simulink model "gm_uz_ninephase_VSD_transformation"  (R2021b)
settings: Solver=FixedStepAuto  StartTime=0.0  StopTime=inf  RelTol=1e-3
undefined symbols (not defined in the file or in its folder): a, b, c
libraries: hdlsllib x90, simulink x32, hdlmdlgenlib x20, dspsigops x7
(part 3 of 6)

== system gm_uz_ninephase_VSD_transformation/abc_to_dq/Divide ==
  in0 : Inport  OutDataTypeStr=fixdt(1, 18, 16)  SampleTime=1e-10
  in1 : Inport  Port=2  OutDataTypeStr=fixdt(1, 27, 16)  SampleTime=1e-10
  globalSchedule : EnablePort  OutDataTypeStr=boolean
  Divide : Product  Inputs=**  OutDataTypeStr=fixdt(1, 27, 16)  SampleTime=1e-10
  HwModeRegister : Delay  DelayLength=double(1)  InitialCondition=0
  HwModeRegister1 : Delay  DelayLength=double(1)  InitialCondition=0
  PipelineRegister : Delay  DelayLength=double(1)  InitialCondition=0
  out0 : Outport  OutDataTypeStr=fixdt(1, 27, 16)  SampleTime=1e-10  InitialOutput=0
  wires:
  PipelineRegister/1 -> out0/1
  in0/1 -> HwModeRegister/1
  in1/1 -> HwModeRegister1/1
  Divide/1 -> PipelineRegister/1
  HwModeRegister/1 -> Divide/1
  HwModeRegister1/1 -> Divide/2

== system gm_uz_ninephase_VSD_transformation/abc_to_dq/Divide1 ==
  in0 : Inport  OutDataTypeStr=fixdt(1, 18, 16)  SampleTime=1e-10
  in1 : Inport  Port=2  OutDataTypeStr=fixdt(1, 27, 16)  SampleTime=1e-10
  globalSchedule : EnablePort  OutDataTypeStr=boolean
  Divide1 : Product  Inputs=**  OutDataTypeStr=fixdt(1, 27, 16)  SampleTime=1e-10
  HwModeRegister : Delay  DelayLength=double(1)  InitialCondition=0
  HwModeRegister1 : Delay  DelayLength=double(1)  InitialCondition=0
  PipelineRegister : Delay  DelayLength=double(1)  InitialCondition=0
  out0 : Outport  OutDataTypeStr=fixdt(1, 27, 16)  SampleTime=1e-10  InitialOutput=0
  wires:
  PipelineRegister/1 -> out0/1
  in0/1 -> HwModeRegister/1
  in1/1 -> HwModeRegister1/1
  Divide1/1 -> PipelineRegister/1
  HwModeRegister/1 -> Divide1/1
  HwModeRegister1/1 -> Divide1/2

== system gm_uz_ninephase_VSD_transformation/abc_to_dq/Divide11 ==
  in0 : Inport  OutDataTypeStr=fixdt(1, 18, 16)  SampleTime=1e-10
  in1 : Inport  Port=2  OutDataTypeStr=fixdt(1, 27, 18)  SampleTime=1e-10
  globalSchedule : EnablePort  OutDataTypeStr=boolean
  Divide1 : Product  Inputs=**  OutDataTypeStr=fixdt(1, 27, 18)  SampleTime=1e-10
  HwModeRegister : Delay  DelayLength=double(1)  InitialCondition=0
  HwModeRegister1 : Delay  DelayLength=double(1)  InitialCondition=0
  PipelineRegister : Delay  DelayLength=double(1)  InitialCondition=0
  out0 : Outport  OutDataTypeStr=fixdt(1, 27, 18)  SampleTime=1e-10  InitialOutput=0
  wires:
  PipelineRegister/1 -> out0/1
  in0/1 -> HwModeRegister/1
  in1/1 -> HwModeRegister1/1
  Divide1/1 -> PipelineRegister/1
  HwModeRegister/1 -> Divide1/1
  HwModeRegister1/1 -> Divide1/2

== system gm_uz_ninephase_VSD_transformation/abc_to_dq/Divide2 ==
  in0 : Inport  OutDataTypeStr=fixdt(1, 18, 16)  SampleTime=1e-10
  in1 : Inport  Port=2  OutDataTypeStr=fixdt(1, 27, 18)  SampleTime=1e-10
  globalSchedule : EnablePort  OutDataTypeStr=boolean
  Divide2 : Product  Inputs=**  OutDataTypeStr=fixdt(1, 27, 18)  SampleTime=1e-10
  HwModeRegister : Delay  DelayLength=double(1)  InitialCondition=0
  HwModeRegister1 : Delay  DelayLength=double(1)  InitialCondition=0
  PipelineRegister : Delay  DelayLength=double(1)  InitialCondition=0
  out0 : Outport  OutDataTypeStr=fixdt(1, 27, 18)  SampleTime=1e-10  InitialOutput=0
  wires:
  PipelineRegister/1 -> out0/1
  in0/1 -> HwModeRegister/1
  in1/1 -> HwModeRegister1/1
  Divide2/1 -> PipelineRegister/1
  HwModeRegister/1 -> Divide2/1
  HwModeRegister1/1 -> Divide2/2

== system gm_uz_ninephase_VSD_transformation/abc_to_dq/Divide21 ==
  in0 : Inport  OutDataTypeStr=fixdt(1, 18, 16)  SampleTime=1e-10
  in1 : Inport  Port=2  OutDataTypeStr=fixdt(1, 27, 16)  SampleTime=1e-10
  globalSchedule : EnablePort  OutDataTypeStr=boolean
  Divide2 : Product  Inputs=**  OutDataTypeStr=fixdt(1, 27, 16)  SampleTime=1e-10
  HwModeRegister : Delay  DelayLength=double(1)  InitialCondition=0
  HwModeRegister1 : Delay  DelayLength=double(1)  InitialCondition=0
  PipelineRegister : Delay  DelayLength=double(1)  InitialCondition=0
  out0 : Outport  OutDataTypeStr=fixdt(1, 27, 16)  SampleTime=1e-10  InitialOutput=0
  wires:
  PipelineRegister/1 -> out0/1
  in0/1 -> HwModeRegister/1
  in1/1 -> HwModeRegister1/1
  Divide2/1 -> PipelineRegister/1
  HwModeRegister/1 -> Divide2/1
  HwModeRegister1/1 -> Divide2/2

== system gm_uz_ninephase_VSD_transformation/abc_to_dq/Divide3 ==
  in0 : Inport  OutDataTypeStr=fixdt(1, 18, 16)  SampleTime=1e-10
  in1 : Inport  Port=2  OutDataTypeStr=fixdt(1, 27, 18)  SampleTime=1e-10
  globalSchedule : EnablePort  OutDataTypeStr=boolean
  Divide3 : Product  Inputs=**  OutDataTypeStr=fixdt(1, 27, 18)  SampleTime=1e-10
  HwModeRegister : Delay  DelayLength=double(1)  InitialCondition=0
  HwModeRegister1 : Delay  DelayLength=double(1)  InitialCondition=0
  PipelineRegister : Delay  DelayLength=double(1)  InitialCondition=0
  out0 : Outport  OutDataTypeStr=fixdt(1, 27, 18)  SampleTime=1e-10  InitialOutput=0
  wires:
  PipelineRegister/1 -> out0/1
  in0/1 -> HwModeRegister/1
  in1/1 -> HwModeRegister1/1
  Divide3/1 -> PipelineRegister/1
  HwModeRegister/1 -> Divide3/1
  HwModeRegister1/1 -> Divide3/2

== system gm_uz_ninephase_VSD_transformation/abc_to_dq/Divide31 ==
  in0 : Inport  OutDataTypeStr=fixdt(1, 18, 16)  SampleTime=1e-10
  in1 : Inport  Port=2  OutDataTypeStr=fixdt(1, 27, 16)  SampleTime=1e-10
  globalSchedule : EnablePort  OutDataTypeStr=boolean
  Divide3 : Product  Inputs=**  OutDataTypeStr=fixdt(1, 27, 16)  SampleTime=1e-10
  HwModeRegister : Delay  DelayLength=double(1)  InitialCondition=0
  HwModeRegister1 : Delay  DelayLength=double(1)  InitialCondition=0
  PipelineRegister : Delay  DelayLength=double(1)  InitialCondition=0
  out0 : Outport  OutDataTypeStr=fixdt(1, 27, 16)  SampleTime=1e-10  InitialOutput=0
  wires:
  PipelineRegister/1 -> out0/1
  in0/1 -> HwModeRegister/1
  in1/1 -> HwModeRegister1/1
  Divide3/1 -> PipelineRegister/1
  HwModeRegister/1 -> Divide3/1
  HwModeRegister1/1 -> Divide3/2

== system gm_uz_ninephase_VSD_transformation/abc_to_dq/Divide4 ==
  in0 : Inport  OutDataTypeStr=fixdt(1, 18, 16)  SampleTime=1e-10
  in1 : Inport  Port=2  OutDataTypeStr=fixdt(1, 27, 18)  SampleTime=1e-10
  globalSchedule : EnablePort  OutDataTypeStr=boolean
  Divide : Product  Inputs=**  OutDataTypeStr=fixdt(1, 27, 18)  SampleTime=1e-10
  HwModeRegister : Delay  DelayLength=double(1)  InitialCondition=0
  HwModeRegister1 : Delay  DelayLength=double(1)  InitialCondition=0
  PipelineRegister : Delay  DelayLength=double(1)  InitialCondition=0
  out0 : Outport  OutDataTypeStr=fixdt(1, 27, 18)  SampleTime=1e-10  InitialOutput=0
  wires:
  PipelineRegister/1 -> out0/1
  in0/1 -> HwModeRegister/1
  in1/1 -> HwModeRegister1/1
  Divide/1 -> PipelineRegister/1
  HwModeRegister/1 -> Divide/1
  HwModeRegister1/1 -> Divide/2

== system gm_uz_ninephase_VSD_transformation/abc_to_dq/Gain ==
  in0 : Inport  OutDataTypeStr=fixdt(1, 18, 19)  SampleTime=1e-10
  in1 : Inport  Port=2  OutDataTypeStr=fixdt(1, 18, 14)  SampleTime=1e-10
  globalSchedule : EnablePort  OutDataTypeStr=boolean
  Gain : Product  Inputs=**  OutDataTypeStr=fixdt(1, 18, 16)  SampleTime=1e-10
  HwModeRegister : Delay  DelayLength=double(1)  InitialCondition=0
  HwModeRegister1 : Delay  DelayLength=double(1)  InitialCondition=0
  PipelineRegister : Delay  DelayLength=double(1)  InitialCondition=0
  out0 : Outport  OutDataTypeStr=fixdt(1, 18, 16)  SampleTime=1e-10  InitialOutput=0
  wires:
  PipelineRegister/1 -> out0/1
  in0/1 -> HwModeRegister/1
  in1/1 -> HwModeRegister1/1
  Gain/1 -> PipelineRegister/1
  HwModeRegister/1 -> Gain/1
  HwModeRegister1/1 -> Gain/2

== system gm_uz_ninephase_VSD_transformation/abc_to_dq/Gain2 ==
  in0 : Inport  OutDataTypeStr=fixdt(1, 27, 16)  PortDimensions=[3]  SampleTime=1e-10
  in1 : Inport  Port=2  OutDataTypeStr=fixdt(1, 18, 16)  SampleTime=1e-10
  globalSchedule : EnablePort  OutDataTypeStr=boolean
  Gain2 : Product  Inputs=**  OutDataTypeStr=fixdt(1, 45, 32)  SampleTime=1e-10
  HwModeRegister : Delay  DelayLength=double(1)  InitialCondition=0
  HwModeRegister1 : Delay  DelayLength=double(1)  InitialCondition=0
  PipelineRegister : Delay  DelayLength=double(1)  InitialCondition=0
  out0 : Outport  OutDataTypeStr=fixdt(1, 45, 32)  PortDimensions=[3]  SampleTime=1e-10  InitialOutput=0
  wires:
  PipelineRegister/1 -> out0/1
  in0/1 -> HwModeRegister/1
  in1/1 -> HwModeRegister1/1
  Gain2/1 -> PipelineRegister/1
  HwModeRegister/1 -> Gain2/1
  HwModeRegister1/1 -> Gain2/2

== system gm_uz_ninephase_VSD_transformation/abc_to_dq/Gain21 ==
  in0 : Inport  OutDataTypeStr=fixdt(1, 27, 16)  PortDimensions=[3]  SampleTime=1e-10
  in1 : Inport  Port=2  OutDataTypeStr=fixdt(1, 18, 16)  SampleTime=1e-10
  globalSchedule : EnablePort  OutDataTypeStr=boolean
  Gain2 : Product  Inputs=**  OutDataTypeStr=fixdt(1, 45, 32)  SampleTime=1e-10
  HwModeRegister : Delay  DelayLength=double(1)  InitialCondition=0
  HwModeRegister1 : Delay  DelayLength=double(1)  InitialCondition=0
  PipelineRegister : Delay  DelayLength=double(1)  InitialCondition=0
  out0 : Outport  OutDataTypeStr=fixdt(1, 45, 32)  PortDimensions=[3]  SampleTime=1e-10  InitialOutput=0
  wires:
  PipelineRegister/1 -> out0/1
  in0/1 -> HwModeRegister/1
  in1/1 -> HwModeRegister1/1
  Gain2/1 -> PipelineRegister/1
  HwModeRegister/1 -> Gain2/1
  HwModeRegister1/1 -> Gain2/2

== system gm_uz_ninephase_VSD_transformation/abc_to_dq/Gain22 ==
  in0 : Inport  OutDataTypeStr=fixdt(1, 27, 16)  PortDimensions=[3]  SampleTime=1e-10
  in1 : Inport  Port=2  OutDataTypeStr=fixdt(1, 18, 16)  SampleTime=1e-10
  globalSchedule : EnablePort  OutDataTypeStr=boolean
  Gain2 : Product  Inputs=**  OutDataTypeStr=fixdt(1, 45, 32)  SampleTime=1e-10
  HwModeRegister : Delay  DelayLength=double(1)  InitialCondition=0
  HwModeRegister1 : Delay  DelayLength=double(1)  InitialCondition=0
  PipelineRegister : Delay  DelayLength=double(1)  InitialCondition=0
  out0 : Outport  OutDataTypeStr=fixdt(1, 45, 32)  PortDimensions=[3]  SampleTime=1e-10  InitialOutput=0
  wires:
  PipelineRegister/1 -> out0/1
  in0/1 -> HwModeRegister/1
  in1/1 -> HwModeRegister1/1
  Gain2/1 -> PipelineRegister/1
  HwModeRegister/1 -> Gain2/1
  HwModeRegister1/1 -> Gain2/2

== system gm_uz_ninephase_VSD_transformation/abc_to_dq/MMul_dot_product ==
  in0 : Inport  OutDataTypeStr=fixdt(1, 18, 16)  PortDimensions=[9 1]  SampleTime=1e-10
  in1 : Inport  Port=2  OutDataTypeStr=fixdt(1, 27, 16)  PortDimensions=[9 1]  SampleTime=1e-10
  globalSchedule : EnablePort  OutDataTypeStr=boolean
  HwModeRegister : Delay  DelayLength=double(1)  InitialCondition=0
  HwModeRegister1 : Delay  DelayLength=double(1)  InitialCondition=0
  MMul_dot_product : Product  Inputs=**  OutDataTypeStr=fixdt(1, 45, 32)  SampleTime=1e-10
  PipelineRegister : Delay  DelayLength=double(1)  InitialCondition=0
  out0 : Outport  OutDataTypeStr=fixdt(1, 45, 32)  PortDimensions=[9 1]  SampleTime=1e-10  InitialOutput=0
  wires:
  PipelineRegister/1 -> out0/1
  in0/1 -> HwModeRegister/1
  in1/1 -> HwModeRegister1/1
  MMul_dot_product/1 -> PipelineRegister/1
  HwModeRegister/1 -> MMul_dot_product/1
  HwModeRegister1/1 -> MMul_dot_product/2

== system gm_uz_ninephase_VSD_transformation/abc_to_dq/MMul_dot_product1 ==
  in0 : Inport  OutDataTypeStr=fixdt(1, 18, 16)  PortDimensions=[9 1]  SampleTime=1e-10
  in1 : Inport  Port=2  OutDataTypeStr=fixdt(1, 27, 16)  PortDimensions=[9 1]  SampleTime=1e-10
  globalSchedule : EnablePort  OutDataTypeStr=boolean
  HwModeRegister : Delay  DelayLength=double(1)  InitialCondition=0
  HwModeRegister1 : Delay  DelayLength=double(1)  InitialCondition=0
  MMul_dot_product : Product  Inputs=**  OutDataTypeStr=fixdt(1, 45, 32)  SampleTime=1e-10
  PipelineRegister : Delay  DelayLength=double(1)  InitialCondition=0
  out0 : Outport  OutDataTypeStr=fixdt(1, 45, 32)  PortDimensions=[9 1]  SampleTime=1e-10  InitialOutput=0
  wires:
  PipelineRegister/1 -> out0/1
  in0/1 -> HwModeRegister/1
  in1/1 -> HwModeRegister1/1
  MMul_dot_product/1 -> PipelineRegister/1
  HwModeRegister/1 -> MMul_dot_product/1
  HwModeRegister1/1 -> MMul_dot_product/2

== system gm_uz_ninephase_VSD_transformation/abc_to_dq/MMul_dot_product2 ==
  in0 : Inport  OutDataTypeStr=fixdt(1, 18, 16)  PortDimensions=[9 1]  SampleTime=1e-10
  in1 : Inport  Port=2  OutDataTypeStr=fixdt(1, 27, 16)  PortDimensions=[9 1]  SampleTime=1e-10
  globalSchedule : EnablePort  OutDataTypeStr=boolean
  HwModeRegister : Delay  DelayLength=double(1)  InitialCondition=0
  HwModeRegister1 : Delay  DelayLength=double(1)  InitialCondition=0
  MMul_dot_product : Product  Inputs=**  OutDataTypeStr=fixdt(1, 45, 32)  SampleTime=1e-10
  PipelineRegister : Delay  DelayLength=double(1)  InitialCondition=0
  out0 : Outport  OutDataTypeStr=fixdt(1, 45, 32)  PortDimensions=[9 1]  SampleTime=1e-10  InitialOutput=0
  wires:
  PipelineRegister/1 -> out0/1
  in0/1 -> HwModeRegister/1
  in1/1 -> HwModeRegister1/1
  MMul_dot_product/1 -> PipelineRegister/1
  HwModeRegister/1 -> MMul_dot_product/1
  HwModeRegister1/1 -> MMul_dot_product/2

== system gm_uz_ninephase_VSD_transformation/abc_to_dq/MMul_dot_product3 ==
  in0 : Inport  OutDataTypeStr=fixdt(1, 18, 16)  PortDimensions=[9 1]  SampleTime=1e-10
  in1 : Inport  Port=2  OutDataTypeStr=fixdt(1, 27, 16)  PortDimensions=[9 1]  SampleTime=1e-10
  globalSchedule : EnablePort  OutDataTypeStr=boolean
  HwModeRegister : Delay  DelayLength=double(1)  InitialCondition=0
  HwModeRegister1 : Delay  DelayLength=double(1)  InitialCondition=0
  MMul_dot_product : Product  Inputs=**  OutDataTypeStr=fixdt(1, 45, 32)  SampleTime=1e-10
  PipelineRegister : Delay  DelayLength=double(1)  InitialCondition=0
  out0 : Outport  OutDataTypeStr=fixdt(1, 45, 32)  PortDimensions=[9 1]  SampleTime=1e-10  InitialOutput=0
  wires:
  PipelineRegister/1 -> out0/1
  in0/1 -> HwModeRegister/1
  in1/1 -> HwModeRegister1/1
  MMul_dot_product/1 -> PipelineRegister/1
  HwModeRegister/1 -> MMul_dot_product/1
  HwModeRegister1/1 -> MMul_dot_product/2

== system gm_uz_ninephase_VSD_transformation/abc_to_dq/MMul_dot_product4 ==
  in0 : Inport  OutDataTypeStr=fixdt(1, 18, 16)  PortDimensions=[9 1]  SampleTime=1e-10
  in1 : Inport  Port=2  OutDataTypeStr=fixdt(1, 27, 16)  PortDimensions=[9 1]  SampleTime=1e-10
  globalSchedule : EnablePort  OutDataTypeStr=boolean
  HwModeRegister : Delay  DelayLength=double(1)  InitialCondition=0
  HwModeRegister1 : Delay  DelayLength=double(1)  InitialCondition=0
  MMul_dot_product : Product  Inputs=**  OutDataTypeStr=fixdt(1, 45, 32)  SampleTime=1e-10
  PipelineRegister : Delay  DelayLength=double(1)  InitialCondition=0
  out0 : Outport  OutDataTypeStr=fixdt(1, 45, 32)  PortDimensions=[9 1]  SampleTime=1e-10  InitialOutput=0
  wires:
  PipelineRegister/1 -> out0/1
  in0/1 -> HwModeRegister/1
  in1/1 -> HwModeRegister1/1
  MMul_dot_product/1 -> PipelineRegister/1
  HwModeRegister/1 -> MMul_dot_product/1
  HwModeRegister1/1 -> MMul_dot_product/2

== system gm_uz_ninephase_VSD_transformation/abc_to_dq/MMul_dot_product5 ==
  in0 : Inport  OutDataTypeStr=fixdt(1, 18, 16)  PortDimensions=[9 1]  SampleTime=1e-10
  in1 : Inport  Port=2  OutDataTypeStr=fixdt(1, 27, 16)  PortDimensions=[9 1]  SampleTime=1e-10
  globalSchedule : EnablePort  OutDataTypeStr=boolean
  HwModeRegister : Delay  DelayLength=double(1)  InitialCondition=0
  HwModeRegister1 : Delay  DelayLength=double(1)  InitialCondition=0
  MMul_dot_product : Product  Inputs=**  OutDataTypeStr=fixdt(1, 45, 32)  SampleTime=1e-10
  PipelineRegister : Delay  DelayLength=double(1)  InitialCondition=0
  out0 : Outport  OutDataTypeStr=fixdt(1, 45, 32)  PortDimensions=[9 1]  SampleTime=1e-10  InitialOutput=0
  wires:
  PipelineRegister/1 -> out0/1
  in0/1 -> HwModeRegister/1
  in1/1 -> HwModeRegister1/1
  MMul_dot_product/1 -> PipelineRegister/1
  HwModeRegister/1 -> MMul_dot_product/1
  HwModeRegister1/1 -> MMul_dot_product/2

== system gm_uz_ninephase_VSD_transformation/abc_to_dq/Product ==
  in0 : Inport  OutDataTypeStr=fixdt(1, 27, 16)  SampleTime=1e-10
  in1 : Inport  Port=2  OutDataTypeStr=fixdt(1, 18, 16)  SampleTime=1e-10
  globalSchedule : EnablePort  OutDataTypeStr=boolean
  HwModeRegister : Delay  DelayLength=double(1)  InitialCondition=0
  HwModeRegister1 : Delay  DelayLength=double(1)  InitialCondition=0
  PipelineRegister : Delay  DelayLength=double(1)  InitialCondition=0
  Product : Product  Inputs=**  OutDataTypeStr=fixdt(1, 27, 16)  SampleTime=1e-10
  out0 : Outport  OutDataTypeStr=fixdt(1, 27, 16)  SampleTime=1e-10  InitialOutput=0
  wires:
  PipelineRegister/1 -> out0/1
  in0/1 -> HwModeRegister/1
  in1/1 -> HwModeRegister1/1
  Product/1 -> PipelineRegister/1
  HwModeRegister/1 -> Product/1
  HwModeRegister1/1 -> Product/2

== system gm_uz_ninephase_VSD_transformation/abc_to_dq/Product1 ==
  in0 : Inport  OutDataTypeStr=fixdt(1, 27, 16)  SampleTime=1e-10
  in1 : Inport  Port=2  OutDataTypeStr=fixdt(1, 18, 16)  SampleTime=1e-10
  globalSchedule : EnablePort  OutDataTypeStr=boolean
  HwModeRegister : Delay  DelayLength=double(1)  InitialCondition=0
  HwModeRegister1 : Delay  DelayLength=double(1)  InitialCondition=0
  PipelineRegister : Delay  DelayLength=double(1)  InitialCondition=0
  Product : Product  Inputs=**  OutDataTypeStr=fixdt(1, 27, 16)  SampleTime=1e-10
  out0 : Outport  OutDataTypeStr=fixdt(1, 27, 16)  SampleTime=1e-10  InitialOutput=0
  wires:
  PipelineRegister/1 -> out0/1
  in0/1 -> HwModeRegister/1
  in1/1 -> HwModeRegister1/1
  Product/1 -> PipelineRegister/1
  HwModeRegister/1 -> Product/1
  HwModeRegister1/1 -> Product/2

== system gm_uz_ninephase_VSD_transformation/abc_to_dq/Product10 ==
  in0 : Inport  OutDataTypeStr=fixdt(1, 27, 16)  SampleTime=1e-10
  in1 : Inport  Port=2  OutDataTypeStr=fixdt(1, 18, 16)  SampleTime=1e-10
  globalSchedule : EnablePort  OutDataTypeStr=boolean
  HwModeRegister : Delay  DelayLength=double(1)  InitialCondition=0
  HwModeRegister1 : Delay  DelayLength=double(1)  InitialCondition=0
  PipelineRegister : Delay  DelayLength=double(1)  InitialCondition=0
  Product : Product  Inputs=**  OutDataTypeStr=fixdt(1, 27, 16)  SampleTime=1e-10
  out0 : Outport  OutDataTypeStr=fixdt(1, 27, 16)  SampleTime=1e-10  InitialOutput=0
  wires:
  PipelineRegister/1 -> out0/1
  in0/1 -> HwModeRegister/1
  in1/1 -> HwModeRegister1/1
  Product/1 -> PipelineRegister/1
  HwModeRegister/1 -> Product/1
  HwModeRegister1/1 -> Product/2

== system gm_uz_ninephase_VSD_transformation/abc_to_dq/Product11 ==
  in0 : Inport  OutDataTypeStr=fixdt(1, 27, 16)  SampleTime=1e-10
  in1 : Inport  Port=2  OutDataTypeStr=fixdt(1, 18, 16)  SampleTime=1e-10
  globalSchedule : EnablePort  OutDataTypeStr=boolean
  HwModeRegister : Delay  DelayLength=double(1)  InitialCondition=0
  HwModeRegister1 : Delay  DelayLength=double(1)  InitialCondition=0
  PipelineRegister : Delay  DelayLength=double(1)  InitialCondition=0
  Product : Product  Inputs=**  OutDataTypeStr=fixdt(1, 27, 16)  SampleTime=1e-10
  out0 : Outport  OutDataTypeStr=fixdt(1, 27, 16)  SampleTime=1e-10  InitialOutput=0
  wires:
  PipelineRegister/1 -> out0/1
  in0/1 -> HwModeRegister/1
  in1/1 -> HwModeRegister1/1
  Product/1 -> PipelineRegister/1
  HwModeRegister/1 -> Product/1
  HwModeRegister1/1 -> Product/2

== system gm_uz_ninephase_VSD_transformation/abc_to_dq/Product2 ==
  in0 : Inport  OutDataTypeStr=fixdt(1, 27, 16)  SampleTime=1e-10
  in1 : Inport  Port=2  OutDataTypeStr=fixdt(1, 18, 16)  SampleTime=1e-10
  globalSchedule : EnablePort  OutDataTypeStr=boolean
  HwModeRegister : Delay  DelayLength=double(1)  InitialCondition=0
  HwModeRegister1 : Delay  DelayLength=double(1)  InitialCondition=0
  PipelineRegister : Delay  DelayLength=double(1)  InitialCondition=0
  Product : Product  Inputs=**  OutDataTypeStr=fixdt(1, 27, 16)  SampleTime=1e-10
  out0 : Outport  OutDataTypeStr=fixdt(1, 27, 16)  SampleTime=1e-10  InitialOutput=0
  wires:
  PipelineRegister/1 -> out0/1
  in0/1 -> HwModeRegister/1
  in1/1 -> HwModeRegister1/1
  Product/1 -> PipelineRegister/1
  HwModeRegister/1 -> Product/1
  HwModeRegister1/1 -> Product/2

== system gm_uz_ninephase_VSD_transformation/abc_to_dq/Product3 ==
  in0 : Inport  OutDataTypeStr=fixdt(1, 27, 16)  SampleTime=1e-10
  in1 : Inport  Port=2  OutDataTypeStr=fixdt(1, 18, 16)  SampleTime=1e-10
  globalSchedule : EnablePort  OutDataTypeStr=boolean
  HwModeRegister : Delay  DelayLength=double(1)  InitialCondition=0
  HwModeRegister1 : Delay  DelayLength=double(1)  InitialCondition=0
  PipelineRegister : Delay  DelayLength=double(1)  InitialCondition=0
  Product : Product  Inputs=**  OutDataTypeStr=fixdt(1, 27, 16)  SampleTime=1e-10
  out0 : Outport  OutDataTypeStr=fixdt(1, 27, 16)  SampleTime=1e-10  InitialOutput=0
  wires:
  PipelineRegister/1 -> out0/1
  in0/1 -> HwModeRegister/1
  in1/1 -> HwModeRegister1/1
  Product/1 -> PipelineRegister/1
  HwModeRegister/1 -> Product/1
  HwModeRegister1/1 -> Product/2

== system gm_uz_ninephase_VSD_transformation/abc_to_dq/Product4 ==
  in0 : Inport  OutDataTypeStr=fixdt(1, 27, 16)  SampleTime=1e-10
  in1 : Inport  Port=2  OutDataTypeStr=fixdt(1, 18, 16)  SampleTime=1e-10
  globalSchedule : EnablePort  OutDataTypeStr=boolean
  HwModeRegister : Delay  DelayLength=double(1)  InitialCondition=0
  HwModeRegister1 : Delay  DelayLength=double(1)  InitialCondition=0
  PipelineRegister : Delay  DelayLength=double(1)  InitialCondition=0
  Product : Product  Inputs=**  OutDataTypeStr=fixdt(1, 27, 16)  SampleTime=1e-10
  out0 : Outport  OutDataTypeStr=fixdt(1, 27, 16)  SampleTime=1e-10  InitialOutput=0
  wires:
  PipelineRegister/1 -> out0/1
  in0/1 -> HwModeRegister/1
  in1/1 -> HwModeRegister1/1
  Product/1 -> PipelineRegister/1
  HwModeRegister/1 -> Product/1
  HwModeRegister1/1 -> Product/2

== system gm_uz_ninephase_VSD_transformation/abc_to_dq/Product5 ==
  in0 : Inport  OutDataTypeStr=fixdt(1, 27, 16)  SampleTime=1e-10
  in1 : Inport  Port=2  OutDataTypeStr=fixdt(1, 18, 16)  SampleTime=1e-10
  globalSchedule : EnablePort  OutDataTypeStr=boolean
  HwModeRegister : Delay  DelayLength=double(1)  InitialCondition=0
  HwModeRegister1 : Delay  DelayLength=double(1)  InitialCondition=0
  PipelineRegister : Delay  DelayLength=double(1)  InitialCondition=0
  Product : Product  Inputs=**  OutDataTypeStr=fixdt(1, 27, 16)  SampleTime=1e-10
  out0 : Outport  OutDataTypeStr=fixdt(1, 27, 16)  SampleTime=1e-10  InitialOutput=0
  wires:
  PipelineRegister/1 -> out0/1
  in0/1 -> HwModeRegister/1
  in1/1 -> HwModeRegister1/1
  Product/1 -> PipelineRegister/1
  HwModeRegister/1 -> Product/1
  HwModeRegister1/1 -> Product/2

== system gm_uz_ninephase_VSD_transformation/abc_to_dq/Product6 ==
  in0 : Inport  OutDataTypeStr=fixdt(1, 27, 16)  SampleTime=1e-10
  in1 : Inport  Port=2  OutDataTypeStr=fixdt(1, 18, 16)  SampleTime=1e-10
  globalSchedule : EnablePort  OutDataTypeStr=boolean
  HwModeRegister : Delay  DelayLength=double(1)  InitialCondition=0
  HwModeRegister1 : Delay  DelayLength=double(1)  InitialCondition=0
  PipelineRegister : Delay  DelayLength=double(1)  InitialCondition=0
  Product : Product  Inputs=**  OutDataTypeStr=fixdt(1, 27, 16)  SampleTime=1e-10
  out0 : Outport  OutDataTypeStr=fixdt(1, 27, 16)  SampleTime=1e-10  InitialOutput=0
  wires:
  PipelineRegister/1 -> out0/1
  in0/1 -> HwModeRegister/1
  in1/1 -> HwModeRegister1/1
  Product/1 -> PipelineRegister/1
  HwModeRegister/1 -> Product/1
  HwModeRegister1/1 -> Product/2

== system gm_uz_ninephase_VSD_transformation/abc_to_dq/Product7 ==
  in0 : Inport  OutDataTypeStr=fixdt(1, 27, 16)  SampleTime=1e-10
  in1 : Inport  Port=2  OutDataTypeStr=fixdt(1, 18, 16)  SampleTime=1e-10
  globalSchedule : EnablePort  OutDataTypeStr=boolean
  HwModeRegister : Delay  DelayLength=double(1)  InitialCondition=0
  HwModeRegister1 : Delay  DelayLength=double(1)  InitialCondition=0
  PipelineRegister : Delay  DelayLength=double(1)  InitialCondition=0
  Product : Product  Inputs=**  OutDataTypeStr=fixdt(1, 27, 16)  SampleTime=1e-10
  out0 : Outport  OutDataTypeStr=fixdt(1, 27, 16)  SampleTime=1e-10  InitialOutput=0
  wires:
  PipelineRegister/1 -> out0/1
  in0/1 -> HwModeRegister/1
  in1/1 -> HwModeRegister1/1
  Product/1 -> PipelineRegister/1
  HwModeRegister/1 -> Product/1
  HwModeRegister1/1 -> Product/2

== system gm_uz_ninephase_VSD_transformation/abc_to_dq/Product8 ==
  in0 : Inport  OutDataTypeStr=fixdt(1, 27, 16)  SampleTime=1e-10
  in1 : Inport  Port=2  OutDataTypeStr=fixdt(1, 18, 16)  SampleTime=1e-10
  globalSchedule : EnablePort  OutDataTypeStr=boolean
  HwModeRegister : Delay  DelayLength=double(1)  InitialCondition=0
  HwModeRegister1 : Delay  DelayLength=double(1)  InitialCondition=0
  PipelineRegister : Delay  DelayLength=double(1)  InitialCondition=0
  Product : Product  Inputs=**  OutDataTypeStr=fixdt(1, 27, 16)  SampleTime=1e-10
  out0 : Outport  OutDataTypeStr=fixdt(1, 27, 16)  SampleTime=1e-10  InitialOutput=0
  wires:
  PipelineRegister/1 -> out0/1
  in0/1 -> HwModeRegister/1
  in1/1 -> HwModeRegister1/1
  Product/1 -> PipelineRegister/1
  HwModeRegister/1 -> Product/1
  HwModeRegister1/1 -> Product/2

== system gm_uz_ninephase_VSD_transformation/abc_to_dq/Product9 ==
  in0 : Inport  OutDataTypeStr=fixdt(1, 27, 16)  SampleTime=1e-10
  in1 : Inport  Port=2  OutDataTypeStr=fixdt(1, 18, 16)  SampleTime=1e-10
  globalSchedule : EnablePort  OutDataTypeStr=boolean
  HwModeRegister : Delay  DelayLength=double(1)  InitialCondition=0
  HwModeRegister1 : Delay  DelayLength=double(1)  InitialCondition=0
  PipelineRegister : Delay  DelayLength=double(1)  InitialCondition=0
  Product : Product  Inputs=**  OutDataTypeStr=fixdt(1, 27, 16)  SampleTime=1e-10
  out0 : Outport  OutDataTypeStr=fixdt(1, 27, 16)  SampleTime=1e-10  InitialOutput=0
  wires:
  PipelineRegister/1 -> out0/1
  in0/1 -> HwModeRegister/1
  in1/1 -> HwModeRegister1/1
  Product/1 -> PipelineRegister/1
  HwModeRegister/1 -> Product/1
  HwModeRegister1/1 -> Product/2

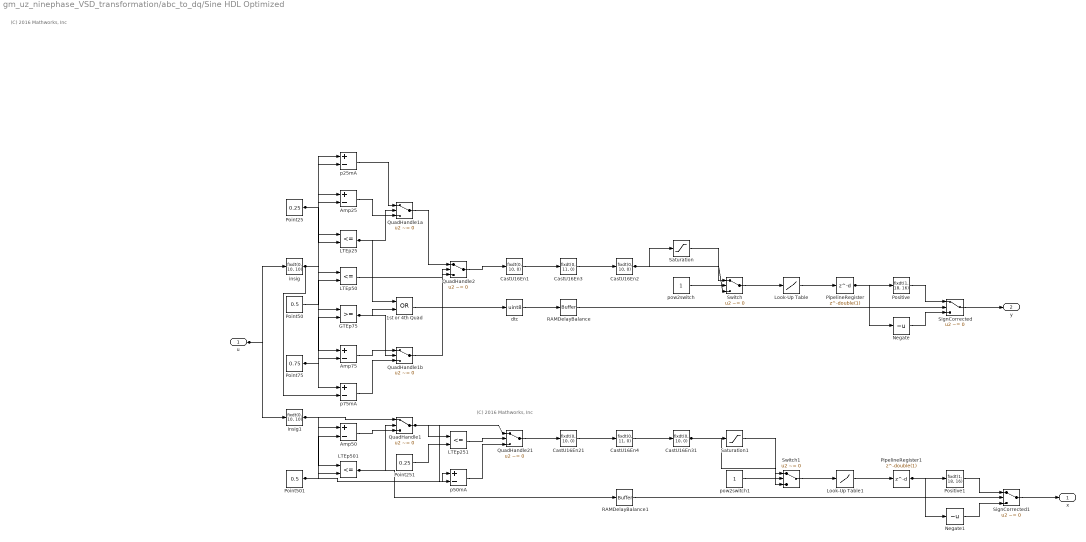
== system gm_uz_ninephase_VSD_transformation/abc_to_dq/Sine HDL Optimized ==
  note: (C) 2016 Mathworks, Inc
  note: (C) 2016 Mathworks, Inc
  u : Inport  OutDataTypeStr=fixdt(1, 18, 16)  SampleTime=1e-10
  1st or 4th Quad : Logic  Operator=OR  AllPortsSameDT=off  OutDataTypeStr=boolean  SampleTime=1e-10
  Amp25 : Sum  Inputs=+-  AccumDataTypeStr=fixdt(1, 19, 18)  OutDataTypeStr=fixdt(1, 19, 18)  SampleTime=1e-10
  Amp50 : Sum  Inputs=+-  AccumDataTypeStr=fixdt(1, 19, 18)  OutDataTypeStr=fixdt(1, 19, 18)  SampleTime=1e-10
  Amp75 : Sum  Inputs=+-  AccumDataTypeStr=fixdt(1, 19, 18)  OutDataTypeStr=fixdt(1, 19, 18)  SampleTime=1e-10
  CastU16En1 : DataTypeConversion  OutDataTypeStr=fixdt(0, 10, 0)  ConvertRealWorld=Stored Integer (SI)  SampleTime=1e-10
  CastU16En2 : DataTypeConversion  OutDataTypeStr=fixdt(0, 10, 0)  ConvertRealWorld=Stored Integer (SI)  SampleTime=1e-10  SaturateOnIntegerOverflow=on
  CastU16En21 : DataTypeConversion  OutDataTypeStr=fixdt(0, 10, 0)  ConvertRealWorld=Stored Integer (SI)  SampleTime=1e-10
  CastU16En3 : DataTypeConversion  OutDataTypeStr=fixdt(0, 11, 0)  SampleTime=1e-10
  CastU16En31 : DataTypeConversion  OutDataTypeStr=fixdt(0, 10, 0)  ConvertRealWorld=Stored Integer (SI)  SampleTime=1e-10  SaturateOnIntegerOverflow=on
  CastU16En4 : DataTypeConversion  OutDataTypeStr=fixdt(0, 11, 0)  SampleTime=1e-10
  GTEp75 : RelationalOperator  OutDataTypeStr=boolean  SampleTime=1e-10  RndMeth=Nearest
  LTEp{25,50,251,501} (4 alike) : RelationalOperator  Operator=<=  OutDataTypeStr=boolean  SampleTime=1e-10  RndMeth=Nearest
  Look-Up Table : Lookup_n-D  NumberOfTableDimensions=1  BreakpointsForDimension1="fi(\"numerictype\",numerictype(0,10,0),\"fimath\",fimath(\"RoundingMethod\", \"Floor\",\"OverflowAction\", \"Wrap\",\"ProductMode\",\"FullPrecision\",\"SumMode\",\"FullPrecision\"),\"Value\",\"[0 1 2 3 4 5 6 7 8 9 10 11 12 13 14 15 16 17 18 19 20 21 22 23 24 25 26 27 28 29 30 31 32 33 34 35 36 37 38 39 40 41 42 43 44 45 46 47 48 49 50 51 52 53 54 55 56 57 58 59 60 61 62 63 64 65 66 67 68 69 70 71 72 73 74 75 76 77 78 79 80 81 82 83 84 85 86 87 88 89 90 91 92 93 94 95 96 97 98 99 100 101 102 103 104 105 106 107 108 109 110 111 112 113 114 115 116 117 118 119 120 121 122 123 124 125 126 127 128 129 130 131 132 133 134 135 136 137 138 139 140 141 142 143 144 145 146 147 148 149 150 151 152 153 154 155 156 157 158 159 160 161 162 163 164 165 166 167 168 169 170 171 172 173 174 175 176 177 178 179 180 181 182 183 184 185 186 187 188 189 190 191 192 193 194 195 196 197 198 199 200 201 202 203 204 205 206 207 208 209 210 211 212 213 214 215 216 217 218 219 220 221 222 223 224 225 226 227 228 229 230 231 232 233 234 235 236 237 238 239 240 241 242 243 244 245 246 247 248 249 250 251 252 253 254 255]\")"  Table="reshape(fi(\"numerictype\",numerictype(1,18,16),\"fimath\",fimath(\"RoundingMethod\", \"Floor\",\"OverflowAction\", \"Wrap\",\"ProductMode\",\"FullPrecision\",\"SumMode\",\"FullPrecision\"),\"Value\",\"[0;0.006134033203125;0.01226806640625;0.018402099609375;0.0245361328125;0.030670166015625;0.03680419921875;0.042938232421875;0.049072265625;0.0551910400390625;0.0613250732421875;0.06744384765625;0.0735626220703125;0.079681396484375;0.0858001708984375;0.0919036865234375;0.0980224609375;0.1041259765625;0.1102294921875;0.1163177490234375;0.122406005859375;0.1284942626953125;0.13458251953125;0.140655517578125;0.146728515625;0.152801513671875;0.1588592529296875;0.1649169921875;0.17095947265625;0.177001953125;0.18304443359375;0.1890716552734375;0.1950836181640625;0.20111083984375;0.2071075439453125;0.213104248046875;0.2191009521484375;0.2250823974609375;0.2310638427734375;0.237030029296875;0.24298095703125;0.248931884765625;0.2548675537109375;0.2607879638671875;0.2667083740234375;0.2726287841796875;0.2785186767578125;0.2844085693359375;0.290283203125;0.2961578369140625;0.302001953125;0.3078460693359375;0.3136749267578125;0.3195037841796875;0.3253173828125;0.3311004638671875;0.336883544921875;0.3426666259765625;0.348419189453125;0.354156494140625;0.359893798828125;0.3656158447265625;0.3713226318359375;0.37701416015625;0.3826904296875;0.3883514404296875;0.3939971923828125;0.399627685546875;0.405242919921875;0.4108428955078125;0.4164276123046875;0.4219970703125;0.42755126953125;0.4330902099609375;0.4386138916015625;0.444122314453125;0.449615478515625;0.455078125;0.460540771484375;0.465972900390625;0.4713897705078125;0.476806640625;0.482177734375;0.487548828125;0.4929046630859375;0.49822998046875;0.5035400390625;0.5088348388671875;0.51409912109375;0.5193634033203125;0.52459716796875;0.5298004150390625;0.535003662109375;0.5401763916015625;0.545318603515625;0.5504608154296875;0.555572509765625;0.5606689453125;0.56573486328125;0.5707855224609375;0.5758056640625;0.580810546875;0.5858001708984375;0.59075927734375;0.595703125;0.600616455078125;0.6055145263671875;0.610382080078125;0.615234375;0.62005615234375;0.6248626708984375;0.629638671875;0.6343994140625;0.639129638671875;0.643829345703125;0.6485137939453125;0.653167724609375;0.657806396484375;0.66241455078125;0.6670074462890625;0.6715545654296875;0.67608642578125;0.68060302734375;0.685089111328125;0.689544677734375;0.6939697265625;0.6983795166015625;0.7027587890625;0.7071075439453125;0.71142578125;0.715728759765625;0.720001220703125;0.7242431640625;0.7284698486328125;0.7326507568359375;0.73681640625;0.7409515380859375;0.74505615234375;0.7491302490234375;0.7531890869140625;0.7572021484375;0.761199951171875;0.765167236328125;0.76910400390625;0.77301025390625;0.776885986328125;0.780731201171875;0.7845611572265625;0.7883453369140625;0.7920989990234375;0.79583740234375;0.799530029296875;0.8032073974609375;0.806854248046875;0.810455322265625;0.8140411376953125;0.8175811767578125;0.82110595703125;0.8245849609375;0.8280487060546875;0.8314666748046875;0.834869384765625;0.838226318359375;0.841552734375;0.8448486328125;0.848114013671875;0.851348876953125;0.85455322265625;0.85772705078125;0.860870361328125;0.8639678955078125;0.8670501708984375;0.870086669921875;0.8730926513671875;0.876068115234375;0.8790130615234375;0.881927490234375;0.884796142578125;0.88763427734375;0.89044189453125;0.893218994140625;0.895965576171875;0.898681640625;0.9013519287109375;0.90399169921875;0.9066009521484375;0.9091644287109375;0.911712646484375;0.914215087890625;0.9166717529296875;0.9191131591796875;0.9215087890625;0.9238739013671875;0.92620849609375;0.9285125732421875;0.9307708740234375;0.9329986572265625;0.9351806640625;0.9373321533203125;0.939453125;0.9415435791015625;0.9435882568359375;0.9456024169921875;0.9475860595703125;0.94952392578125;0.9514312744140625;0.95330810546875;0.95513916015625;0.956939697265625;0.958709716796875;0.9604339599609375;0.962127685546875;0.963775634765625;0.96539306640625;0.96697998046875;0.9685211181640625;0.97003173828125;0.97149658203125;0.9729461669921875;0.974334716796875;0.9757080078125;0.9770355224609375;0.9783172607421875;0.9795684814453125;0.9807891845703125;0.981964111328125 ...(+541 chars)]\"), [1  256])"  InterpMethod=Flat  ExtrapMethod=Clip  DiagnosticForOutOfRangeInput=Error  SampleTime=1e-10  OutDataTypeStr=fixdt(1, 18, 16)  InputSameDT=on
  Look-Up Table1 : Lookup_n-D  NumberOfTableDimensions=1  BreakpointsForDimension1="fi(\"numerictype\",numerictype(0,10,0),\"fimath\",fimath(\"RoundingMethod\", \"Floor\",\"OverflowAction\", \"Wrap\",\"ProductMode\",\"FullPrecision\",\"SumMode\",\"FullPrecision\"),\"Value\",\"[0 1 2 3 4 5 6 7 8 9 10 11 12 13 14 15 16 17 18 19 20 21 22 23 24 25 26 27 28 29 30 31 32 33 34 35 36 37 38 39 40 41 42 43 44 45 46 47 48 49 50 51 52 53 54 55 56 57 58 59 60 61 62 63 64 65 66 67 68 69 70 71 72 73 74 75 76 77 78 79 80 81 82 83 84 85 86 87 88 89 90 91 92 93 94 95 96 97 98 99 100 101 102 103 104 105 106 107 108 109 110 111 112 113 114 115 116 117 118 119 120 121 122 123 124 125 126 127 128 129 130 131 132 133 134 135 136 137 138 139 140 141 142 143 144 145 146 147 148 149 150 151 152 153 154 155 156 157 158 159 160 161 162 163 164 165 166 167 168 169 170 171 172 173 174 175 176 177 178 179 180 181 182 183 184 185 186 187 188 189 190 191 192 193 194 195 196 197 198 199 200 201 202 203 204 205 206 207 208 209 210 211 212 213 214 215 216 217 218 219 220 221 222 223 224 225 226 227 228 229 230 231 232 233 234 235 236 237 238 239 240 241 242 243 244 245 246 247 248 249 250 251 252 253 254 255]\")"  Table="reshape(fi(\"numerictype\",numerictype(1,18,16),\"fimath\",fimath(\"RoundingMethod\", \"Floor\",\"OverflowAction\", \"Wrap\",\"ProductMode\",\"FullPrecision\",\"SumMode\",\"FullPrecision\"),\"Value\",\"[0;0.006134033203125;0.01226806640625;0.018402099609375;0.0245361328125;0.030670166015625;0.03680419921875;0.042938232421875;0.049072265625;0.0551910400390625;0.0613250732421875;0.06744384765625;0.0735626220703125;0.079681396484375;0.0858001708984375;0.0919036865234375;0.0980224609375;0.1041259765625;0.1102294921875;0.1163177490234375;0.122406005859375;0.1284942626953125;0.13458251953125;0.140655517578125;0.146728515625;0.152801513671875;0.1588592529296875;0.1649169921875;0.17095947265625;0.177001953125;0.18304443359375;0.1890716552734375;0.1950836181640625;0.20111083984375;0.2071075439453125;0.213104248046875;0.2191009521484375;0.2250823974609375;0.2310638427734375;0.237030029296875;0.24298095703125;0.248931884765625;0.2548675537109375;0.2607879638671875;0.2667083740234375;0.2726287841796875;0.2785186767578125;0.2844085693359375;0.290283203125;0.2961578369140625;0.302001953125;0.3078460693359375;0.3136749267578125;0.3195037841796875;0.3253173828125;0.3311004638671875;0.336883544921875;0.3426666259765625;0.348419189453125;0.354156494140625;0.359893798828125;0.3656158447265625;0.3713226318359375;0.37701416015625;0.3826904296875;0.3883514404296875;0.3939971923828125;0.399627685546875;0.405242919921875;0.4108428955078125;0.4164276123046875;0.4219970703125;0.42755126953125;0.4330902099609375;0.4386138916015625;0.444122314453125;0.449615478515625;0.455078125;0.460540771484375;0.465972900390625;0.4713897705078125;0.476806640625;0.482177734375;0.487548828125;0.4929046630859375;0.49822998046875;0.5035400390625;0.5088348388671875;0.51409912109375;0.5193634033203125;0.52459716796875;0.5298004150390625;0.535003662109375;0.5401763916015625;0.545318603515625;0.5504608154296875;0.555572509765625;0.5606689453125;0.56573486328125;0.5707855224609375;0.5758056640625;0.580810546875;0.5858001708984375;0.59075927734375;0.595703125;0.600616455078125;0.6055145263671875;0.610382080078125;0.615234375;0.62005615234375;0.6248626708984375;0.629638671875;0.6343994140625;0.639129638671875;0.643829345703125;0.6485137939453125;0.653167724609375;0.657806396484375;0.66241455078125;0.6670074462890625;0.6715545654296875;0.67608642578125;0.68060302734375;0.685089111328125;0.689544677734375;0.6939697265625;0.6983795166015625;0.7027587890625;0.7071075439453125;0.71142578125;0.715728759765625;0.720001220703125;0.7242431640625;0.7284698486328125;0.7326507568359375;0.73681640625;0.7409515380859375;0.74505615234375;0.7491302490234375;0.7531890869140625;0.7572021484375;0.761199951171875;0.765167236328125;0.76910400390625;0.77301025390625;0.776885986328125;0.780731201171875;0.7845611572265625;0.7883453369140625;0.7920989990234375;0.79583740234375;0.799530029296875;0.8032073974609375;0.806854248046875;0.810455322265625;0.8140411376953125;0.8175811767578125;0.82110595703125;0.8245849609375;0.8280487060546875;0.8314666748046875;0.834869384765625;0.838226318359375;0.841552734375;0.8448486328125;0.848114013671875;0.851348876953125;0.85455322265625;0.85772705078125;0.860870361328125;0.8639678955078125;0.8670501708984375;0.870086669921875;0.8730926513671875;0.876068115234375;0.8790130615234375;0.881927490234375;0.884796142578125;0.88763427734375;0.89044189453125;0.893218994140625;0.895965576171875;0.898681640625;0.9013519287109375;0.90399169921875;0.9066009521484375;0.9091644287109375;0.911712646484375;0.914215087890625;0.9166717529296875;0.9191131591796875;0.9215087890625;0.9238739013671875;0.92620849609375;0.9285125732421875;0.9307708740234375;0.9329986572265625;0.9351806640625;0.9373321533203125;0.939453125;0.9415435791015625;0.9435882568359375;0.9456024169921875;0.9475860595703125;0.94952392578125;0.9514312744140625;0.95330810546875;0.95513916015625;0.956939697265625;0.958709716796875;0.9604339599609375;0.962127685546875;0.963775634765625;0.96539306640625;0.96697998046875;0.9685211181640625;0.97003173828125;0.97149658203125;0.9729461669921875;0.974334716796875;0.9757080078125;0.9770355224609375;0.9783172607421875;0.9795684814453125;0.9807891845703125;0.981964111328125 ...(+541 chars)]\"), [1  256])"  InterpMethod=Flat  ExtrapMethod=Clip  DiagnosticForOutOfRangeInput=Error  SampleTime=1e-10  OutDataTypeStr=fixdt(1, 18, 16)  InputSameDT=on
  Negate : UnaryMinus  SampleTime=1e-10
  Negate1 : UnaryMinus  SampleTime=1e-10
  PipelineRegister : Delay  DelayLength=double(1)  InitialCondition=0  SampleTime=1e-10
  PipelineRegister1 : Delay  DelayLength=double(1)  InitialCondition=0  SampleTime=1e-10
  Point25 : Constant  Value=0.25  OutDataTypeStr=fixdt(0, 18, 18)  SampleTime=1e-10
  Point251 : Constant  Value=0.25  OutDataTypeStr=fixdt(0, 18, 18)  SampleTime=1e-10
  Point50 : Constant  Value=0.5  OutDataTypeStr=fixdt(0, 18, 18)  SampleTime=1e-10
  Point501 : Constant  Value=0.5  OutDataTypeStr=fixdt(0, 18, 18)  SampleTime=1e-10
  Point75 : Constant  Value=0.75  OutDataTypeStr=fixdt(0, 18, 18)  SampleTime=1e-10
  Positive : DataTypeConversion  OutDataTypeStr=fixdt(1, 18, 16)  SampleTime=1e-10
  Positive1 : DataTypeConversion  OutDataTypeStr=fixdt(1, 18, 16)  SampleTime=1e-10
  QuadHandle1 : Switch  Criteria=u2 ~= 0  Threshold=double(0)  OutDataTypeStr=fixdt(1, 19, 18)  SampleTime=1e-10
  QuadHandle1a : Switch  Criteria=u2 ~= 0  Threshold=double(0)  OutDataTypeStr=fixdt(1, 19, 18)  SampleTime=1e-10
  QuadHandle1b : Switch  Criteria=u2 ~= 0  Threshold=double(0)  OutDataTypeStr=fixdt(1, 19, 18)  SampleTime=1e-10
  QuadHandle2 : Switch  Criteria=u2 ~= 0  Threshold=double(0)  OutDataTypeStr=fixdt(0, 10, 10)  SampleTime=1e-10  SaturateOnIntegerOverflow=on
  QuadHandle21 : Switch  Criteria=u2 ~= 0  Threshold=double(0)  OutDataTypeStr=fixdt(0, 10, 10)  SampleTime=1e-10
  RAMDelayBalance : hdlmdlgenlib/Buffer
      settings: SourceProductBaseCode=SL
  RAMDelayBalance1 : hdlmdlgenlib/Buffer
      settings: SourceProductBaseCode=SL
  Saturation : Saturate  UpperLimit="fi(0,0,10,0,\"hex\",\"0ff\")"  LowerLimit="fi(0,0,10,0,\"hex\",\"000\")"  SampleTime=1e-10  OutDataTypeStr=fixdt(0, 10, 0)
  Saturation1 : Saturate  UpperLimit="fi(0,0,10,0,\"hex\",\"0ff\")"  LowerLimit="fi(0,0,10,0,\"hex\",\"000\")"  SampleTime=1e-10  OutDataTypeStr=fixdt(0, 10, 0)
  SignCorrected : Switch  Criteria=u2 ~= 0  Threshold=double(0)  OutDataTypeStr=fixdt(1, 18, 16)  SampleTime=1e-10
  SignCorrected1 : Switch  Criteria=u2 ~= 0  Threshold=double(0)  OutDataTypeStr=fixdt(1, 18, 16)  SampleTime=1e-10
  Switch : Switch  Criteria=u2 ~= 0  Threshold=double(0)  OutDataTypeStr=fixdt(0, 10, 0)  SampleTime=1e-10
  Switch1 : Switch  Criteria=u2 ~= 0  Threshold=double(0)  OutDataTypeStr=fixdt(0, 10, 0)  SampleTime=1e-10
  dtc : DataTypeConversion  OutDataTypeStr=uint8  SampleTime=1e-10
  insig : DataTypeConversion  OutDataTypeStr=fixdt(0, 10, 10)  SampleTime=1e-10
  insig1 : DataTypeConversion  OutDataTypeStr=fixdt(0, 10, 10)  SampleTime=1e-10
  p25mA : Sum  Inputs=+-  AccumDataTypeStr=fixdt(1, 19, 18)  OutDataTypeStr=fixdt(1, 19, 18)  SampleTime=1e-10
  p50mA : Sum  Inputs=+-  AccumDataTypeStr=fixdt(1, 20, 18)  OutDataTypeStr=fixdt(1, 20, 18)  SampleTime=1e-10
  p75mA : Sum  Inputs=+-  AccumDataTypeStr=fixdt(1, 19, 18)  OutDataTypeStr=fixdt(1, 19, 18)  SampleTime=1e-10
  pow2switch : Constant  OutDataTypeStr=boolean  SampleTime=1e-10
  pow2switch1 : Constant  OutDataTypeStr=boolean  SampleTime=1e-10
  x : Outport  SampleTime=1e-10
  y : Outport  Port=2  SampleTime=1e-10
  wires:
  dtc/1 -> RAMDelayBalance/1
  Amp25/1 -> QuadHandle1a/3
  Amp75/1 -> QuadHandle1b/1
  CastU16En1/1 -> CastU16En3/1
  CastU16En2/1 -> Switch/3, Saturation/1
  CastU16En3/1 -> CastU16En2/1
  GTEp75/1 -> QuadHandle1b/2, 1st or 4th Quad/2
  LTEp25/1 -> QuadHandle1a/2, 1st or 4th Quad/1
  LTEp50/1 -> QuadHandle2/2
  PipelineRegister/1 -> Positive/1, Negate/1
  Negate/1 -> SignCorrected/3
  Point25/1 -> p25mA/1, LTEp25/2, Amp25/2
  Point50/1 -> LTEp50/2
  Point75/1 -> p75mA/1, GTEp75/2, Amp75/2
  Positive/1 -> SignCorrected/1
  QuadHandle1a/1 -> QuadHandle2/1
  QuadHandle1b/1 -> QuadHandle2/3
  QuadHandle2/1 -> CastU16En1/1
  Saturation/1 -> Switch/1
  SignCorrected/1 -> y/1
  Switch/1 -> Look-Up Table/1
  insig/1 -> p75mA/2, p25mA/2, LTEp50/1, LTEp25/1, GTEp75/1, Amp75/1, Amp25/1
  p25mA/1 -> QuadHandle1a/1
  p75mA/1 -> QuadHandle1b/3
  pow2switch/1 -> Switch/2
  Amp50/1 -> QuadHandle1/3
  CastU16En21/1 -> CastU16En4/1
  CastU16En31/1 -> Switch1/3, Saturation1/1
  CastU16En4/1 -> CastU16En31/1
  LTEp251/1 -> QuadHandle21/2
  LTEp501/1 -> QuadHandle1/2, RAMDelayBalance1/1
  PipelineRegister1/1 -> Positive1/1, Negate1/1
  Negate1/1 -> SignCorrected1/3
  Point251/1 -> LTEp251/2
  Point501/1 -> p50mA/1, LTEp501/2, Amp50/2
  Positive1/1 -> SignCorrected1/1
  QuadHandle1/1 -> p50mA/2, QuadHandle21/1, LTEp251/1
  QuadHandle21/1 -> CastU16En21/1
  Saturation1/1 -> Switch1/1
  SignCorrected1/1 -> x/1
  Switch1/1 -> Look-Up Table1/1
  insig1/1 -> QuadHandle1/1, LTEp501/1, Amp50/1
  p50mA/1 -> QuadHandle21/3
  pow2switch1/1 -> Switch1/2
  1st or 4th Quad/1 -> dtc/1
  RAMDelayBalance1/1 -> SignCorrected1/2
  RAMDelayBalance/1 -> SignCorrected/2
  u/1 -> insig1/1, insig/1
  Look-Up Table/1 -> PipelineRegister/1
  Look-Up Table1/1 -> PipelineRegister1/1

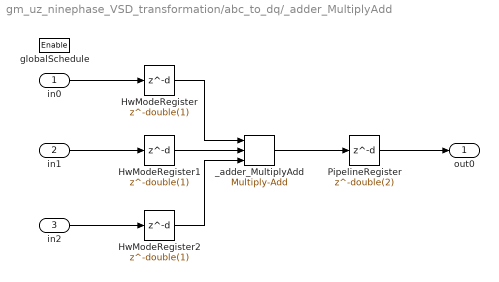
== system gm_uz_ninephase_VSD_transformation/abc_to_dq/_adder_MultiplyAdd ==
  in0 : Inport  OutDataTypeStr=fixdt(1, 18, 17)  SampleTime=1e-10
  in1 : Inport  Port=2  OutDataTypeStr=fixdt(1, 27, 16)  SampleTime=1e-10
  in2 : Inport  Port=3  OutDataTypeStr=fixdt(1, 27, 16)  SampleTime=1e-10
  globalSchedule : EnablePort  OutDataTypeStr=boolean
  HwModeRegister : Delay  DelayLength=double(1)  InitialCondition=0
  HwModeRegister1 : Delay  DelayLength=double(1)  InitialCondition=0
  HwModeRegister2 : Delay  DelayLength=double(1)  InitialCondition=0
  PipelineRegister : Delay  DelayLength=double(2)  InitialCondition=0
  _adder_MultiplyAdd : hdlsllib/HDL Operations/Multiply-Add  Function=c+(a.*b)  datatype=fixdt(1, 46, 33)  DoSatur=off  FMA=off
      settings: SourceProductBaseCode=SL
  out0 : Outport  OutDataTypeStr=fixdt(1, 46, 33)  SampleTime=1e-10  InitialOutput=0
  wires:
  PipelineRegister/1 -> out0/1
  in0/1 -> HwModeRegister/1
  in1/1 -> HwModeRegister1/1
  in2/1 -> HwModeRegister2/1
  _adder_MultiplyAdd/1 -> PipelineRegister/1
  HwModeRegister/1 -> _adder_MultiplyAdd/1
  HwModeRegister1/1 -> _adder_MultiplyAdd/2
  HwModeRegister2/1 -> _adder_MultiplyAdd/3

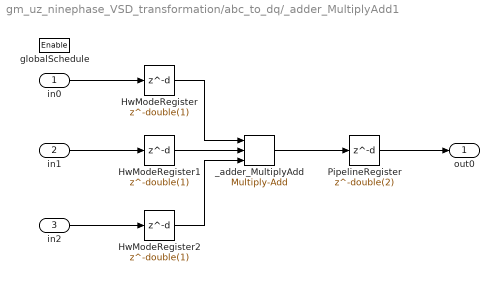
== system gm_uz_ninephase_VSD_transformation/abc_to_dq/_adder_MultiplyAdd1 ==
  in0 : Inport  OutDataTypeStr=fixdt(1, 18, 17)  SampleTime=1e-10
  in1 : Inport  Port=2  OutDataTypeStr=fixdt(1, 27, 16)  SampleTime=1e-10
  in2 : Inport  Port=3  OutDataTypeStr=fixdt(1, 27, 16)  SampleTime=1e-10
  globalSchedule : EnablePort  OutDataTypeStr=boolean
  HwModeRegister : Delay  DelayLength=double(1)  InitialCondition=0
  HwModeRegister1 : Delay  DelayLength=double(1)  InitialCondition=0
  HwModeRegister2 : Delay  DelayLength=double(1)  InitialCondition=0
  PipelineRegister : Delay  DelayLength=double(2)  InitialCondition=0
  _adder_MultiplyAdd : hdlsllib/HDL Operations/Multiply-Add  Function=c+(a.*b)  datatype=fixdt(1, 46, 33)  DoSatur=off  FMA=off
      settings: SourceProductBaseCode=SL
  out0 : Outport  OutDataTypeStr=fixdt(1, 46, 33)  SampleTime=1e-10  InitialOutput=0
  wires:
  PipelineRegister/1 -> out0/1
  in0/1 -> HwModeRegister/1
  in1/1 -> HwModeRegister1/1
  in2/1 -> HwModeRegister2/1
  _adder_MultiplyAdd/1 -> PipelineRegister/1
  HwModeRegister/1 -> _adder_MultiplyAdd/1
  HwModeRegister1/1 -> _adder_MultiplyAdd/2
  HwModeRegister2/1 -> _adder_MultiplyAdd/3

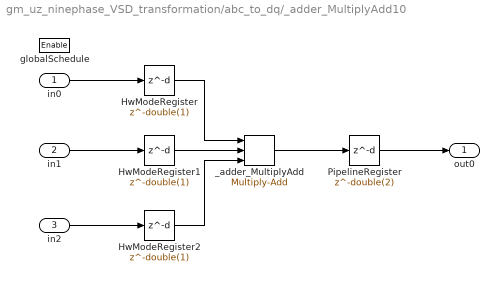
== system gm_uz_ninephase_VSD_transformation/abc_to_dq/_adder_MultiplyAdd10 ==
  in0 : Inport  OutDataTypeStr=fixdt(1, 18, 17)  SampleTime=1e-10
  in1 : Inport  Port=2  OutDataTypeStr=fixdt(1, 27, 16)  SampleTime=1e-10
  in2 : Inport  Port=3  OutDataTypeStr=fixdt(1, 27, 16)  SampleTime=1e-10
  globalSchedule : EnablePort  OutDataTypeStr=boolean
  HwModeRegister : Delay  DelayLength=double(1)  InitialCondition=0
  HwModeRegister1 : Delay  DelayLength=double(1)  InitialCondition=0
  HwModeRegister2 : Delay  DelayLength=double(1)  InitialCondition=0
  PipelineRegister : Delay  DelayLength=double(2)  InitialCondition=0
  _adder_MultiplyAdd : hdlsllib/HDL Operations/Multiply-Add  Function=c+(a.*b)  datatype=fixdt(1, 46, 33)  DoSatur=off  FMA=off
      settings: SourceProductBaseCode=SL
  out0 : Outport  OutDataTypeStr=fixdt(1, 46, 33)  SampleTime=1e-10  InitialOutput=0
  wires:
  PipelineRegister/1 -> out0/1
  in0/1 -> HwModeRegister/1
  in1/1 -> HwModeRegister1/1
  in2/1 -> HwModeRegister2/1
  _adder_MultiplyAdd/1 -> PipelineRegister/1
  HwModeRegister/1 -> _adder_MultiplyAdd/1
  HwModeRegister1/1 -> _adder_MultiplyAdd/2
  HwModeRegister2/1 -> _adder_MultiplyAdd/3

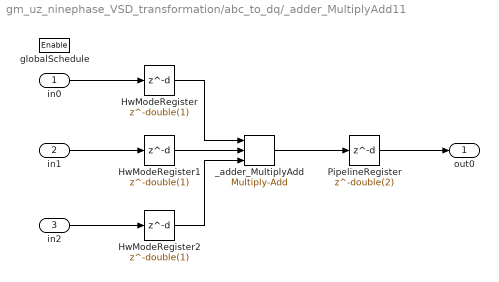
== system gm_uz_ninephase_VSD_transformation/abc_to_dq/_adder_MultiplyAdd11 ==
  in0 : Inport  OutDataTypeStr=fixdt(1, 18, 17)  SampleTime=1e-10
  in1 : Inport  Port=2  OutDataTypeStr=fixdt(1, 27, 16)  SampleTime=1e-10
  in2 : Inport  Port=3  OutDataTypeStr=fixdt(1, 27, 16)  SampleTime=1e-10
  globalSchedule : EnablePort  OutDataTypeStr=boolean
  HwModeRegister : Delay  DelayLength=double(1)  InitialCondition=0
  HwModeRegister1 : Delay  DelayLength=double(1)  InitialCondition=0
  HwModeRegister2 : Delay  DelayLength=double(1)  InitialCondition=0
  PipelineRegister : Delay  DelayLength=double(2)  InitialCondition=0
  _adder_MultiplyAdd : hdlsllib/HDL Operations/Multiply-Add  Function=c+(a.*b)  datatype=fixdt(1, 46, 33)  DoSatur=off  FMA=off
      settings: SourceProductBaseCode=SL
  out0 : Outport  OutDataTypeStr=fixdt(1, 46, 33)  SampleTime=1e-10  InitialOutput=0
  wires:
  PipelineRegister/1 -> out0/1
  in0/1 -> HwModeRegister/1
  in1/1 -> HwModeRegister1/1
  in2/1 -> HwModeRegister2/1
  _adder_MultiplyAdd/1 -> PipelineRegister/1
  HwModeRegister/1 -> _adder_MultiplyAdd/1
  HwModeRegister1/1 -> _adder_MultiplyAdd/2
  HwModeRegister2/1 -> _adder_MultiplyAdd/3
